simulink model "CONTROL_CARTESIAN"  (R2019b)
settings: Solver=VariableStepAuto  StartTime=0.0  StopTime=10.0  RelTol=1e-3
undefined symbols (not defined in the file): gain_planar_2R, q0_planar_2R, time_step
settings Model: Creator=simone  LastModifiedBy=simone

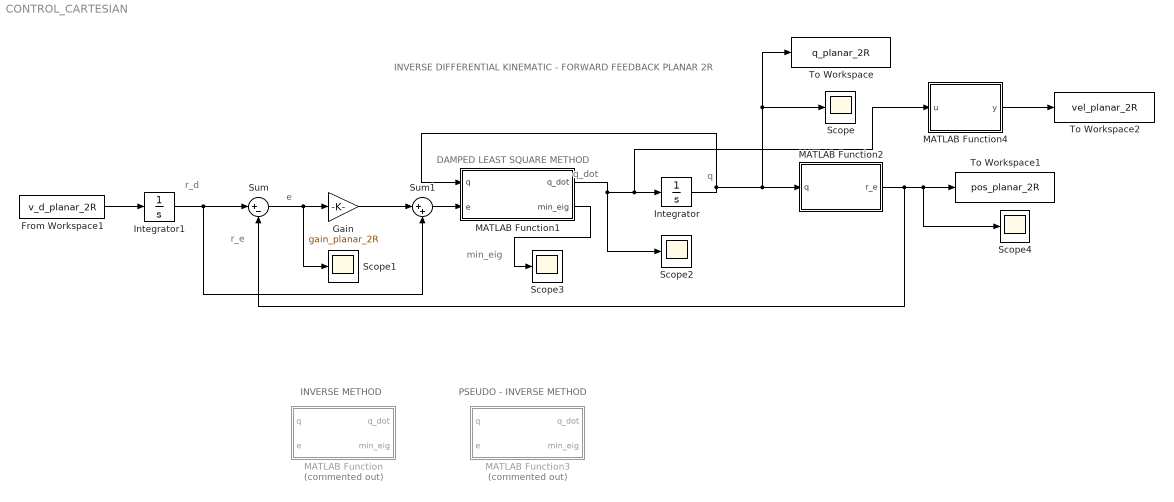
== system CONTROL_CARTESIAN ==
  note: e
  note: q_dot
  note: INVERSE DIFFERENTIAL KINEMATIC - FORWARD FEEDBACK
      | PLANAR 2R
  note: DAMPED LEAST SQUARE METHOD
  note: PSEUDO - INVERSE METHOD
  note: q
  note: r_d
  note: INVERSE METHOD
  note: r_e
  note: min_eig
  From Workspace1 : FromWorkspace  VariableName=v_d_planar_2R  SampleTime=time_step
  Gain : Gain  Gain=gain_planar_2R
  Integrator : Integrator  InitialCondition=q0_planar_2R
  Integrator1 : Integrator  InitialCondition=q0_planar_2R
  MATLAB Function : MATLAB Function  Commented=on  TreatAsAtomicUnit=on
  MATLAB Function1 : MATLAB Function  TreatAsAtomicUnit=on
  MATLAB Function2 : MATLAB Function  TreatAsAtomicUnit=on
  MATLAB Function3 : MATLAB Function  Commented=on  TreatAsAtomicUnit=on
  MATLAB Function4 : MATLAB Function  TreatAsAtomicUnit=on
  Scope{,1..4} (5 alike) : Scope
  Sum : Sum  Inputs=|+-
  Sum1 : Sum  Inputs=|++
  To Workspace : ToWorkspace  VariableName=q_planar_2R  SaveFormat=Timeseries  SampleTime=time_step
  To Workspace1 : ToWorkspace  VariableName=pos_planar_2R  SaveFormat=Timeseries  SampleTime=time_step
  To Workspace2 : ToWorkspace  VariableName=vel_planar_2R  SaveFormat=Timeseries  SampleTime=time_step
  wires:
  MATLAB Function2/1(r_e) -> Sum/2, Scope4/1, To Workspace1/1
  Integrator/1 -> MATLAB Function1/1(q), To Workspace/1, Scope/1, MATLAB Function2/1(q)
  Sum1/1 -> MATLAB Function1/2(e)
  MATLAB Function1/1(q_dot) -> Scope2/1, MATLAB Function4/1(u), Integrator/1
  Gain/1 -> Sum1/1
  Sum/1 -> Scope1/1, Gain/1
  MATLAB Function1/2(min_eig) -> Scope3/1
  Integrator1/1 -> Sum1/2, Sum/1
  From Workspace1/1 -> Integrator1/1
  MATLAB Function4/1(y) -> To Workspace2/1

== matlab function CONTROL_CARTESIAN/MATLAB Function1 ==
  data: q_dot output; q input; e input; min_eig output
function [q_dot,min_eig] = J_dls(q,e)
J_q = [-sin(q(1)+q(2))-sin(q(1)) -sin(q(1)+q(2));
    cos(q(1)+q(2))+cos(q(1)) cos(q(1)+q(2))];
min_eig = abs(min(eig(J_q)));
q_dot = J_q\e;
if min_eig < 1e-1
    lamb = 0.1;
    J_q = SR_ROBO.dls_jacobian(J_q,lamb);
    min_eig = abs(min(eig(J_q)));
    q_dot = J_q*e;
end
end

== matlab function CONTROL_CARTESIAN/MATLAB Function ==
  data: q_dot output; q input; e input; min_eig output
function [q_dot,min_eig] = J_r(q,e)
J_q = [-sin(q(1)+q(2))-sin(q(1)) -sin(q(1)+q(2));
    cos(q(1)+q(2))+cos(q(1)) cos(q(1)+q(2))];
min_eig = abs(min(eig(J_q)));
q_dot = J_q\e;

== matlab function CONTROL_CARTESIAN/MATLAB Function2 ==
  data: r_e output; q input
function r_e = F_r(q)
%PLANAR ROBOT (2R)
r_e = [cos(q(1)+q(2))+cos(q(1));
    sin(q(1)+q(2))+sin(q(1))];

== matlab function CONTROL_CARTESIAN/MATLAB Function3 ==
  data: q_dot output; q input; e input; min_eig output
function [q_dot,min_eig] = J_dls(q,e)
J_q = [-sin(q(1)+q(2))-sin(q(1)) -sin(q(1)+q(2));
    cos(q(1)+q(2))+cos(q(1)) cos(q(1)+q(2))];
min_eig = abs(min(eig(J_q)));

J_psed = SR_ROBO.pseudo_inverse_jacobian(J_q);

q_dot = J_psed*e;

== matlab function CONTROL_CARTESIAN/MATLAB Function4 ==
  data: u input; y output
function y = fcn(u)

y = u;
